simulink model "kinovaMicoSimscapeModel"  (R2021b)
settings: Solver=VariableStepAuto  StartTime=0.0  StopTime=0.3  FixedStep=0.01  RelTol=1e-3
PostLoadFcn:
  | micoRigidBodyTreeCreation;
  | IC=deg2rad([-90,180,180,0,0,0]);
  | interactiveHomePosition=deg2rad([-90 90 177.5 90 0 0]');
  | load("./KinovaMicoSimscapeVariantConfigurations.mat");
values from neighbouring files (symbols this model uses):
  micoCandlePosition = deg2rad([0,180,180,0,0,0])    [KinovaMicoSimscapeInitializeScript.m]    (also in generatingRandomTrajectory.m)
  ViaPointsTaskSpace = [ViaPointsTaskSpace;[[pi;0;pi],[pi;0;pi],[pi;0;pi],[pi;0;pi],[0;0;0],[0;0;0],[pi;0;pi]]]    [KinovaMicoSimscapeInitializeScript.m]    (also in generatingRandomTrajectory.m = [ViaPointsTaskSpace;zeros(3,7)])
undefined symbols (not defined in the file or in its folder): Mico, ViaPointsJointSpace, X, Y, Z
libraries: sm_lib x26, nesl_utility x19, robotcorelib x4, robotmaniplib x3, pid_lib x2
(part 49 of 50)

== matlab function kinovaMicoSimscapeModel/Variant Subsystem/TaskSpaceController/Sliding Robust Task Space Control/dJdt ==
  data: q input; dJdt output; dq input
function dJdt = fcn(q,dq)
q1=q(1);
q2=q(2);
q3=q(3);
q4=q(4);
q5=q(5);

dq1=dq(1);
dq2=dq(2);
dq3=dq(3);
dq4=dq(4);
dq5=dq(5);

dJdt1_1 = 0.14155926623698178445920348167419*sin(q5)*(cos(q4)*(dq1*cos(q1)*cos(q2)*cos(q3) + dq1*cos(q1)*sin(q2)*sin(q3) + dq2*cos(q2)*sin(q1)*sin(q3) - 1.0*dq2*cos(q3)*sin(q1)*sin(q2) - 1.0*dq3*cos(q2)*sin(q1)*sin(q3) + dq3*cos(q3)*sin(q1)*sin(q2)) - 1.0*dq4*sin(q4)*(sin(q1)*sin(q2)*sin(q3) + cos(q2)*cos(q3)*sin(q1)) + dq4*cos(q1)*cos(q4) - 1.0*dq1*sin(q1)*sin(q4)) - 0.14484150251703908907074946910143*sin(q4)*(dq1*cos(q1)*cos(q2)*cos(q3) + dq1*cos(q1)*sin(q2)*sin(q3) + dq2*cos(q2)*sin(q1)*sin(q3) - 1.0*dq2*cos(q3)*sin(q1)*sin(q2) - 1.0*dq3*cos(q2)*sin(q1)*sin(q3) + dq3*cos(q3)*sin(q1)*sin(q2)) - 0.12259392070255614726193016394973*cos(q5)*(dq1*cos(q1)*cos(q2)*sin(q3) - 1.0*dq1*cos(q1)*cos(q3)*sin(q2) - 1.0*dq2*cos(q2)*cos(q3)*sin(q1) + dq3*cos(q2)*cos(q3)*sin(q1) - 1.0*dq2*sin(q1)*sin(q2)*sin(q3) + dq3*sin(q1)*sin(q2)*sin(q3)) + 0.0069999999999996731503415503539145*dq1*sin(q1) + 0.070779633118078777442860882729292*cos(q5)*(sin(q4)*(dq1*cos(q1)*cos(q2)*cos(q3) + dq1*cos(q1)*sin(q2)*sin(q3) + dq2*cos(q2)*sin(q1)*sin(q3) - 1.0*dq2*cos(q3)*sin(q1)*sin(q2) - 1.0*dq3*cos(q2)*sin(q1)*sin(q3) + dq3*cos(q3)*sin(q1)*sin(q2)) + dq1*cos(q4)*sin(q1) + dq4*cos(q1)*sin(q4) + dq4*cos(q4)*(sin(q1)*sin(q2)*sin(q3) + cos(q2)*cos(q3)*sin(q1))) + 0.12259392070255614726193016394973*dq5*sin(q5)*(cos(q2)*sin(q1)*sin(q3) - 1.0*cos(q3)*sin(q1)*sin(q2)) - 0.29000000000002046363078989088535*dq1*cos(q1)*sin(q2) - 0.29000000000002046363078989088535*dq2*cos(q2)*sin(q1) - 0.14484150251703908907074946910143*dq1*cos(q4)*sin(q1) - 0.14484150251703908907074946910143*dq4*cos(q1)*sin(q4) + 0.14155926623698178445920348167419*dq5*cos(q5)*(cos(q1)*sin(q4) + cos(q4)*(sin(q1)*sin(q2)*sin(q3) + cos(q2)*cos(q3)*sin(q1))) + 0.070779633118078777442860882729292*dq5*sin(q5)*(cos(q1)*cos(q4) - 1.0*sin(q4)*(sin(q1)*sin(q2)*sin(q3) + cos(q2)*cos(q3)*sin(q1))) - 0.14484150251703908907074946910143*dq4*cos(q4)*(sin(q1)*sin(q2)*sin(q3) + cos(q2)*cos(q3)*sin(q1)) - 0.24948499999945283889246638864279*dq1*cos(q1)*cos(q2)*sin(q3) + 0.24948499999945283889246638864279*dq1*cos(q1)*cos(q3)*sin(q2) + 0.24948499999945283889246638864279*dq2*cos(q2)*cos(q3)*sin(q1) - 0.24948499999945283889246638864279*dq3*cos(q2)*cos(q3)*sin(q1) + 0.24948499999945283889246638864279*dq2*sin(q1)*sin(q2)*sin(q3) - 0.24948499999945283889246638864279*dq3*sin(q1)*sin(q2)*sin(q3);
dJdt1_2 = 0.12259392070255614726193016394973*cos(q5)*(dq1*cos(q2)*cos(q3)*sin(q1) - 1.0*dq2*cos(q1)*cos(q2)*sin(q3) + dq2*cos(q1)*cos(q3)*sin(q2) + dq3*cos(q1)*cos(q2)*sin(q3) - 1.0*dq3*cos(q1)*cos(q3)*sin(q2) + dq1*sin(q1)*sin(q2)*sin(q3)) - 0.14484150251703908907074946910143*sin(q4)*(dq2*cos(q1)*cos(q2)*cos(q3) - 1.0*dq3*cos(q1)*cos(q2)*cos(q3) + dq1*cos(q2)*sin(q1)*sin(q3) - 1.0*dq1*cos(q3)*sin(q1)*sin(q2) + dq2*cos(q1)*sin(q2)*sin(q3) - 1.0*dq3*cos(q1)*sin(q2)*sin(q3)) + 0.14484150251703908907074946910143*dq4*cos(q4)*(cos(q1)*cos(q2)*sin(q3) - 1.0*cos(q1)*cos(q3)*sin(q2)) + 0.14155926623698178445920348167419*cos(q4)*sin(q5)*(dq2*cos(q1)*cos(q2)*cos(q3) - 1.0*dq3*cos(q1)*cos(q2)*cos(q3) + dq1*cos(q2)*sin(q1)*sin(q3) - 1.0*dq1*cos(q3)*sin(q1)*sin(q2) + dq2*cos(q1)*sin(q2)*sin(q3) - 1.0*dq3*cos(q1)*sin(q2)*sin(q3)) + 0.070779633118078777442860882729292*cos(q5)*sin(q4)*(dq2*cos(q1)*cos(q2)*cos(q3) - 1.0*dq3*cos(q1)*cos(q2)*cos(q3) + dq1*cos(q2)*sin(q1)*sin(q3) - 1.0*dq1*cos(q3)*sin(q1)*sin(q2) + dq2*cos(q1)*sin(q2)*sin(q3) - 1.0*dq3*cos(q1)*sin(q2)*sin(q3)) - 0.29000000000002046363078989088535*dq1*cos(q2)*sin(q1) - 0.29000000000002046363078989088535*dq2*cos(q1)*sin(q2) + 0.12259392070255614726193016394973*dq5*sin(q5)*(cos(q1)*cos(q2)*cos(q3) + cos(q1)*sin(q2)*sin(q3)) + 0.14155926623698178445920348167419*dq4*sin(q4)*sin(q5)*(cos(q1)*cos(q2)*sin(q3) - 1.0*cos(q1)*cos(q3)*sin(q2)) + 0.070779633118078777442860882729292*dq5*sin(q4)*sin(q5)*(cos(q1)*cos(q2)*sin(q3) - 1.0*cos(q1)*cos(q3)*sin(q2)) + 0.24948499999945283889246638864279*dq1*cos(q2)*cos(q3)*sin(q1) - 0.24948499999945283889246638864279*dq2*cos(q1)*cos(q2)*sin(q3) + 0.24948499999945283889246638864279*dq2*cos(q1)*cos(q3)*sin(q2) + 0.24948499999945283889246638864279*dq3*cos(q1)*cos(q2)*sin(q3) - 0.24948499999945283889246638864279*dq3*cos(q1)*cos(q3)*sin(q2) + 0.24948499999945283889246638864279*dq1*sin(q1)*sin(q2)*sin(q3) - 0.070779633118078777442860882729292*dq4*cos(q4)*cos(q5)*(cos(q1)*cos(q2)*sin(q3) - 1.0*cos(q1)*cos(q3)*sin(q2)) - 0.14155926623698178445920348167419*dq5*cos(q4)*cos(q5)*(cos(q1)*cos(q2)*sin(q3) - 1.0*cos(q1)*cos(q3)*sin(q2));
dJdt1_3 = 0.14484150251703908907074946910143*sin(q4)*(dq2*cos(q1)*cos(q2)*cos(q3) - 1.0*dq3*cos(q1)*cos(q2)*cos(q3) + dq1*cos(q2)*sin(q1)*sin(q3) - 1.0*dq1*cos(q3)*sin(q1)*sin(q2) + dq2*cos(q1)*sin(q2)*sin(q3) - 1.0*dq3*cos(q1)*sin(q2)*sin(q3)) - 0.12259392070255614726193016394973*cos(q5)*(dq1*cos(q2)*cos(q3)*sin(q1) - 1.0*dq2*cos(q1)*cos(q2)*sin(q3) + dq2*cos(q1)*cos(q3)*sin(q2) + dq3*cos(q1)*cos(q2)*sin(q3) - 1.0*dq3*cos(q1)*cos(q3)*sin(q2) + dq1*sin(q1)*sin(q2)*sin(q3)) - 0.14484150251703908907074946910143*dq4*cos(q4)*(cos(q1)*cos(q2)*sin(q3) - 1.0*cos(q1)*cos(q3)*sin(q2)) - 0.14155926623698178445920348167419*cos(q4)*sin(q5)*(dq2*cos(q1)*cos(q2)*cos(q3) - 1.0*dq3*cos(q1)*cos(q2)*cos(q3) + dq1*cos(q2)*sin(q1)*sin(q3) - 1.0*dq1*cos(q3)*sin(q1)*sin(q2) + dq2*cos(q1)*sin(q2)*sin(q3) - 1.0*dq3*cos(q1)*sin(q2)*sin(q3)) - 0.070779633118078777442860882729292*cos(q5)*sin(q4)*(dq2*cos(q1)*cos(q2)*cos(q3) - 1.0*dq3*cos(q1)*cos(q2)*cos(q3) + dq1*cos(q2)*sin(q1)*sin(q3) - 1.0*dq1*cos(q3)*sin(q1)*sin(q2) + dq2*cos(q1)*sin(q2)*sin(q3) - 1.0*dq3*cos(q1)*sin(q2)*sin(q3)) - 0.12259392070255614726193016394973*dq5*sin(q5)*(cos(q1)*cos(q2)*cos(q3) + cos(q1)*sin(q2)*sin(q3)) - 0.14155926623698178445920348167419*dq4*sin(q4)*sin(q5)*(cos(q1)*cos(q2)*sin(q3) - 1.0*cos(q1)*cos(q3)*sin(q2)) - 0.070779633118078777442860882729292*dq5*sin(q4)*sin(q5)*(cos(q1)*cos(q2)*sin(q3) - 1.0*cos(q1)*cos(q3)*sin(q2)) - 0.24948499999945283889246638864279*dq1*cos(q2)*cos(q3)*sin(q1) + 0.24948499999945283889246638864279*dq2*cos(q1)*cos(q2)*sin(q3) - 0.24948499999945283889246638864279*dq2*cos(q1)*cos(q3)*sin(q2) - 0.24948499999945283889246638864279*dq3*cos(q1)*cos(q2)*sin(q3) + 0.24948499999945283889246638864279*dq3*cos(q1)*cos(q3)*sin(q2) - 0.24948499999945283889246638864279*dq1*sin(q1)*sin(q2)*sin(q3) + 0.070779633118078777442860882729292*dq4*cos(q4)*cos(q5)*(cos(q1)*cos(q2)*sin(q3) - 1.0*cos(q1)*cos(q3)*sin(q2)) + 0.14155926623698178445920348167419*dq5*cos(q4)*cos(q5)*(cos(q1)*cos(q2)*sin(q3) - 1.0*cos(q1)*cos(q3)*sin(q2));
dJdt1_4 = 0.070779633118078777442860882729292*cos(q5)*(cos(q4)*(dq1*cos(q2)*cos(q3)*sin(q1) - 1.0*dq2*cos(q1)*cos(q2)*sin(q3) + dq2*cos(q1)*cos(q3)*sin(q2) + dq3*cos(q1)*cos(q2)*sin(q3) - 1.0*dq3*cos(q1)*cos(q3)*sin(q2) + dq1*sin(q1)*sin(q2)*sin(q3)) + dq1*cos(q1)*sin(q4) + dq4*cos(q4)*sin(q1) + dq4*sin(q4)*(cos(q1)*cos(q2)*cos(q3) + cos(q1)*sin(q2)*sin(q3))) - 0.14484150251703908907074946910143*cos(q4)*(dq1*cos(q2)*cos(q3)*sin(q1) - 1.0*dq2*cos(q1)*cos(q2)*sin(q3) + dq2*cos(q1)*cos(q3)*sin(q2) + dq3*cos(q1)*cos(q2)*sin(q3) - 1.0*dq3*cos(q1)*cos(q3)*sin(q2) + dq1*sin(q1)*sin(q2)*sin(q3)) - 0.14155926623698178445920348167419*sin(q5)*(sin(q4)*(dq1*cos(q2)*cos(q3)*sin(q1) - 1.0*dq2*cos(q1)*cos(q2)*sin(q3) + dq2*cos(q1)*cos(q3)*sin(q2) + dq3*cos(q1)*cos(q2)*sin(q3) - 1.0*dq3*cos(q1)*cos(q3)*sin(q2) + dq1*sin(q1)*sin(q2)*sin(q3)) - 1.0*dq1*cos(q1)*cos(q4) + dq4*sin(q1)*sin(q4) - 1.0*dq4*cos(q4)*(cos(q1)*cos(q2)*cos(q3) + cos(q1)*sin(q2)*sin(q3))) - 0.14484150251703908907074946910143*dq1*cos(q1)*sin(q4) - 0.14484150251703908907074946910143*dq4*cos(q4)*sin(q1) + 0.14155926623698178445920348167419*dq5*cos(q5)*(cos(q4)*sin(q1) + sin(q4)*(cos(q1)*cos(q2)*cos(q3) + cos(q1)*sin(q2)*sin(q3))) - 0.070779633118078777442860882729292*dq5*sin(q5)*(sin(q1)*sin(q4) - 1.0*cos(q4)*(cos(q1)*cos(q2)*cos(q3) + cos(q1)*sin(q2)*sin(q3))) - 0.14484150251703908907074946910143*dq4*sin(q4)*(cos(q1)*cos(q2)*cos(q3) + cos(q1)*sin(q2)*sin(q3));
dJdt1_5 = 0.12259392070255614726193016394973*sin(q5)*(dq2*cos(q1)*cos(q2)*cos(q3) - 1.0*dq3*cos(q1)*cos(q2)*cos(q3) + dq1*cos(q2)*sin(q1)*sin(q3) - 1.0*dq1*cos(q3)*sin(q1)*sin(q2) + dq2*cos(q1)*sin(q2)*sin(q3) - 1.0*dq3*cos(q1)*sin(q2)*sin(q3)) - 0.070779633118078777442860882729292*sin(q5)*(sin(q4)*(dq1*cos(q2)*cos(q3)*sin(q1) - 1.0*dq2*cos(q1)*cos(q2)*sin(q3) + dq2*cos(q1)*cos(q3)*sin(q2) + dq3*cos(q1)*cos(q2)*sin(q3) - 1.0*dq3*cos(q1)*cos(q3)*sin(q2) + dq1*sin(q1)*sin(q2)*sin(q3)) - 1.0*dq1*cos(q1)*cos(q4) + dq4*sin(q1)*sin(q4) - 1.0*dq4*cos(q4)*(cos(q1)*cos(q2)*cos(q3) + cos(q1)*sin(q2)*sin(q3))) + 0.14155926623698178445920348167419*cos(q5)*(cos(q4)*(dq1*cos(q2)*cos(q3)*sin(q1) - 1.0*dq2*cos(q1)*cos(q2)*sin(q3) + dq2*cos(q1)*cos(q3)*sin(q2) + dq3*cos(q1)*cos(q2)*sin(q3) - 1.0*dq3*cos(q1)*cos(q3)*sin(q2) + dq1*sin(q1)*sin(q2)*sin(q3)) + dq1*cos(q1)*sin(q4) + dq4*cos(q4)*sin(q1) + dq4*sin(q4)*(cos(q1)*cos(q2)*cos(q3) + cos(q1)*sin(q2)*sin(q3))) - 0.12259392070255614726193016394973*dq5*cos(q5)*(cos(q1)*cos(q2)*sin(q3) - 1.0*cos(q1)*cos(q3)*sin(q2)) + 0.070779633118078777442860882729292*dq5*cos(q5)*(cos(q4)*sin(q1) + sin(q4)*(cos(q1)*cos(q2)*cos(q3) + cos(q1)*sin(q2)*sin(q3))) - 0.14155926623698178445920348167419*dq5*sin(q5)*(sin(q1)*sin(q4) - 1.0*cos(q4)*(cos(q1)*cos(q2)*cos(q3) + cos(q1)*sin(q2)*sin(q3)));
dJdt1_6 = 0.0;
dJdt2_1 = 0.14484150251703908907074946910143*sin(q4)*(dq1*cos(q2)*cos(q3)*sin(q1) - 1.0*dq2*cos(q1)*cos(q2)*sin(q3) + dq2*cos(q1)*cos(q3)*sin(q2) + dq3*cos(q1)*cos(q2)*sin(q3) - 1.0*dq3*cos(q1)*cos(q3)*sin(q2) + dq1*sin(q1)*sin(q2)*sin(q3)) - 0.070779633118078777442860882729292*cos(q5)*(sin(q4)*(dq1*cos(q2)*cos(q3)*sin(q1) - 1.0*dq2*cos(q1)*cos(q2)*sin(q3) + dq2*cos(q1)*cos(q3)*sin(q2) + dq3*cos(q1)*cos(q2)*sin(q3) - 1.0*dq3*cos(q1)*cos(q3)*sin(q2) + dq1*sin(q1)*sin(q2)*sin(q3)) - 1.0*dq1*cos(q1)*cos(q4) + dq4*sin(q1)*sin(q4) - 1.0*dq4*cos(q4)*(cos(q1)*cos(q2)*cos(q3) + cos(q1)*sin(q2)*sin(q3))) + 0.12259392070255614726193016394973*cos(q5)*(dq2*cos(q1)*cos(q2)*cos(q3) - 1.0*dq3*cos(q1)*cos(q2)*cos(q3) + dq1*cos(q2)*sin(q1)*sin(q3) - 1.0*dq1*cos(q3)*sin(q1)*sin(q2) + dq2*cos(q1)*sin(q2)*sin(q3) - 1.0*dq3*cos(q1)*sin(q2)*sin(q3)) - 0.14155926623698178445920348167419*sin(q5)*(cos(q4)*(dq1*cos(q2)*cos(q3)*sin(q1) - 1.0*dq2*cos(q1)*cos(q2)*sin(q3) + dq2*cos(q1)*cos(q3)*sin(q2) + dq3*cos(q1)*cos(q2)*sin(q3) - 1.0*dq3*cos(q1)*cos(q3)*sin(q2) + dq1*sin(q1)*sin(q2)*sin(q3)) + dq1*cos(q1)*sin(q4) + dq4*cos(q4)*sin(q1) + dq4*sin(q4)*(cos(q1)*cos(q2)*cos(q3) + cos(q1)*sin(q2)*sin(q3))) + 0.0069999999999996731503415503539145*dq1*cos(q1) + 0.12259392070255614726193016394973*dq5*sin(q5)*(cos(q1)*cos(q2)*sin(q3) - 1.0*cos(q1)*cos(q3)*sin(q2)) - 0.29000000000002046363078989088535*dq2*cos(q1)*cos(q2) - 0.14484150251703908907074946910143*dq1*cos(q1)*cos(q4) + 0.29000000000002046363078989088535*dq1*sin(q1)*sin(q2) + 0.14484150251703908907074946910143*dq4*sin(q1)*sin(q4) - 0.070779633118078777442860882729292*dq5*sin(q5)*(cos(q4)*sin(q1) + sin(q4)*(cos(q1)*cos(q2)*cos(q3) + cos(q1)*sin(q2)*sin(q3))) - 0.14155926623698178445920348167419*dq5*cos(q5)*(sin(q1)*sin(q4) - 1.0*cos(q4)*(cos(q1)*cos(q2)*cos(q3) + cos(q1)*sin(q2)*sin(q3))) - 0.14484150251703908907074946910143*dq4*cos(q4)*(cos(q1)*cos(q2)*cos(q3) + cos(q1)*sin(q2)*sin(q3)) + 0.24948499999945283889246638864279*dq2*cos(q1)*cos(q2)*cos(q3) - 0.24948499999945283889246638864279*dq3*cos(q1)*cos(q2)*cos(q3) + 0.24948499999945283889246638864279*dq1*cos(q2)*sin(q1)*sin(q3) - 0.24948499999945283889246638864279*dq1*cos(q3)*sin(q1)*sin(q2) + 0.24948499999945283889246638864279*dq2*cos(q1)*sin(q2)*sin(q3) - 0.24948499999945283889246638864279*dq3*cos(q1)*sin(q2)*sin(q3);
dJdt2_2 = 0.12259392070255614726193016394973*cos(q5)*(dq1*cos(q1)*cos(q2)*cos(q3) + dq1*cos(q1)*sin(q2)*sin(q3) + dq2*cos(q2)*sin(q1)*sin(q3) - 1.0*dq2*cos(q3)*sin(q1)*sin(q2) - 1.0*dq3*cos(q2)*sin(q1)*sin(q3) + dq3*cos(q3)*sin(q1)*sin(q2)) - 0.14484150251703908907074946910143*sin(q4)*(dq1*cos(q1)*cos(q2)*sin(q3) - 1.0*dq1*cos(q1)*cos(q3)*sin(q2) - 1.0*dq2*cos(q2)*cos(q3)*sin(q1) + dq3*cos(q2)*cos(q3)*sin(q1) - 1.0*dq2*sin(q1)*sin(q2)*sin(q3) + dq3*sin(q1)*sin(q2)*sin(q3)) - 0.12259392070255614726193016394973*dq5*sin(q5)*(sin(q1)*sin(q2)*sin(q3) + cos(q2)*cos(q3)*sin(q1)) - 0.14484150251703908907074946910143*dq4*cos(q4)*(cos(q2)*sin(q1)*sin(q3) - 1.0*cos(q3)*sin(q1)*sin(q2)) + 0.14155926623698178445920348167419*cos(q4)*sin(q5)*(dq1*cos(q1)*cos(q2)*sin(q3) - 1.0*dq1*cos(q1)*cos(q3)*sin(q2) - 1.0*dq2*cos(q2)*cos(q3)*sin(q1) + dq3*cos(q2)*cos(q3)*sin(q1) - 1.0*dq2*sin(q1)*sin(q2)*sin(q3) + dq3*sin(q1)*sin(q2)*sin(q3)) + 0.070779633118078777442860882729292*cos(q5)*sin(q4)*(dq1*cos(q1)*cos(q2)*sin(q3) - 1.0*dq1*cos(q1)*cos(q3)*sin(q2) - 1.0*dq2*cos(q2)*cos(q3)*sin(q1) + dq3*cos(q2)*cos(q3)*sin(q1) - 1.0*dq2*sin(q1)*sin(q2)*sin(q3) + dq3*sin(q1)*sin(q2)*sin(q3)) - 0.29000000000002046363078989088535*dq1*cos(q1)*cos(q2) + 0.29000000000002046363078989088535*dq2*sin(q1)*sin(q2) + 0.070779633118078777442860882729292*dq4*cos(q4)*cos(q5)*(cos(q2)*sin(q1)*sin(q3) - 1.0*cos(q3)*sin(q1)*sin(q2)) + 0.14155926623698178445920348167419*dq5*cos(q4)*cos(q5)*(cos(q2)*sin(q1)*sin(q3) - 1.0*cos(q3)*sin(q1)*sin(q2)) - 0.14155926623698178445920348167419*dq4*sin(q4)*sin(q5)*(cos(q2)*sin(q1)*sin(q3) - 1.0*cos(q3)*sin(q1)*sin(q2)) - 0.070779633118078777442860882729292*dq5*sin(q4)*sin(q5)*(cos(q2)*sin(q1)*sin(q3) - 1.0*cos(q3)*sin(q1)*sin(q2)) + 0.24948499999945283889246638864279*dq1*cos(q1)*cos(q2)*cos(q3) + 0.24948499999945283889246638864279*dq1*cos(q1)*sin(q2)*sin(q3) + 0.24948499999945283889246638864279*dq2*cos(q2)*sin(q1)*sin(q3) - 0.24948499999945283889246638864279*dq2*cos(q3)*sin(q1)*sin(q2) - 0.24948499999945283889246638864279*dq3*cos(q2)*sin(q1)*sin(q3) + 0.24948499999945283889246638864279*dq3*cos(q3)*sin(q1)*sin(q2);
dJdt2_3 = 0.14484150251703908907074946910143*sin(q4)*(dq1*cos(q1)*cos(q2)*sin(q3) - 1.0*dq1*cos(q1)*cos(q3)*sin(q2) - 1.0*dq2*cos(q2)*cos(q3)*sin(q1) + dq3*cos(q2)*cos(q3)*sin(q1) - 1.0*dq2*sin(q1)*sin(q2)*sin(q3) + dq3*sin(q1)*sin(q2)*sin(q3)) - 0.12259392070255614726193016394973*cos(q5)*(dq1*cos(q1)*cos(q2)*cos(q3) + dq1*cos(q1)*sin(q2)*sin(q3) + dq2*cos(q2)*sin(q1)*sin(q3) - 1.0*dq2*cos(q3)*sin(q1)*sin(q2) - 1.0*dq3*cos(q2)*sin(q1)*sin(q3) + dq3*cos(q3)*sin(q1)*sin(q2)) + 0.12259392070255614726193016394973*dq5*sin(q5)*(sin(q1)*sin(q2)*sin(q3) + cos(q2)*cos(q3)*sin(q1)) + 0.14484150251703908907074946910143*dq4*cos(q4)*(cos(q2)*sin(q1)*sin(q3) - 1.0*cos(q3)*sin(q1)*sin(q2)) - 0.14155926623698178445920348167419*cos(q4)*sin(q5)*(dq1*cos(q1)*cos(q2)*sin(q3) - 1.0*dq1*cos(q1)*cos(q3)*sin(q2) - 1.0*dq2*cos(q2)*cos(q3)*sin(q1) + dq3*cos(q2)*cos(q3)*sin(q1) - 1.0*dq2*sin(q1)*sin(q2)*sin(q3) + dq3*sin(q1)*sin(q2)*sin(q3)) - 0.070779633118078777442860882729292*cos(q5)*sin(q4)*(dq1*cos(q1)*cos(q2)*sin(q3) - 1.0*dq1*cos(q1)*cos(q3)*sin(q2) - 1.0*dq2*cos(q2)*cos(q3)*sin(q1) + dq3*cos(q2)*cos(q3)*sin(q1) - 1.0*dq2*sin(q1)*sin(q2)*sin(q3) + dq3*sin(q1)*sin(q2)*sin(q3)) - 0.070779633118078777442860882729292*dq4*cos(q4)*cos(q5)*(cos(q2)*sin(q1)*sin(q3) - 1.0*cos(q3)*sin(q1)*sin(q2)) - 0.14155926623698178445920348167419*dq5*cos(q4)*cos(q5)*(cos(q2)*sin(q1)*sin(q3) - 1.0*cos(q3)*sin(q1)*sin(q2)) + 0.14155926623698178445920348167419*dq4*sin(q4)*sin(q5)*(cos(q2)*sin(q1)*sin(q3) - 1.0*cos(q3)*sin(q1)*sin(q2)) + 0.070779633118078777442860882729292*dq5*sin(q4)*sin(q5)*(cos(q2)*sin(q1)*sin(q3) - 1.0*cos(q3)*sin(q1)*sin(q2)) - 0.24948499999945283889246638864279*dq1*cos(q1)*cos(q2)*cos(q3) - 0.24948499999945283889246638864279*dq1*cos(q1)*sin(q2)*sin(q3) - 0.24948499999945283889246638864279*dq2*cos(q2)*sin(q1)*sin(q3) + 0.24948499999945283889246638864279*dq2*cos(q3)*sin(q1)*sin(q2) + 0.24948499999945283889246638864279*dq3*cos(q2)*sin(q1)*sin(q3) - 0.24948499999945283889246638864279*dq3*cos(q3)*sin(q1)*sin(q2);
dJdt2_4 = 0.070779633118078777442860882729292*cos(q5)*(cos(q4)*(dq1*cos(q1)*cos(q2)*cos(q3) + dq1*cos(q1)*sin(q2)*sin(q3) + dq2*cos(q2)*sin(q1)*sin(q3) - 1.0*dq2*cos(q3)*sin(q1)*sin(q2) - 1.0*dq3*cos(q2)*sin(q1)*sin(q3) + dq3*cos(q3)*sin(q1)*sin(q2)) - 1.0*dq4*sin(q4)*(sin(q1)*sin(q2)*sin(q3) + cos(q2)*cos(q3)*sin(q1)) + dq4*cos(q1)*cos(q4) - 1.0*dq1*sin(q1)*sin(q4)) - 0.14484150251703908907074946910143*cos(q4)*(dq1*cos(q1)*cos(q2)*cos(q3) + dq1*cos(q1)*sin(q2)*sin(q3) + dq2*cos(q2)*sin(q1)*sin(q3) - 1.0*dq2*cos(q3)*sin(q1)*sin(q2) - 1.0*dq3*cos(q2)*sin(q1)*sin(q3) + dq3*cos(q3)*sin(q1)*sin(q2)) - 0.14155926623698178445920348167419*sin(q5)*(sin(q4)*(dq1*cos(q1)*cos(q2)*cos(q3) + dq1*cos(q1)*sin(q2)*sin(q3) + dq2*cos(q2)*sin(q1)*sin(q3) - 1.0*dq2*cos(q3)*sin(q1)*sin(q2) - 1.0*dq3*cos(q2)*sin(q1)*sin(q3) + dq3*cos(q3)*sin(q1)*sin(q2)) + dq1*cos(q4)*sin(q1) + dq4*cos(q1)*sin(q4) + dq4*cos(q4)*(sin(q1)*sin(q2)*sin(q3) + cos(q2)*cos(q3)*sin(q1))) + 0.14484150251703908907074946910143*dq4*sin(q4)*(sin(q1)*sin(q2)*sin(q3) + cos(q2)*cos(q3)*sin(q1)) - 0.14484150251703908907074946910143*dq4*cos(q1)*cos(q4) + 0.14484150251703908907074946910143*dq1*sin(q1)*sin(q4) - 0.070779633118078777442860882729292*dq5*sin(q5)*(cos(q1)*sin(q4) + cos(q4)*(sin(q1)*sin(q2)*sin(q3) + cos(q2)*cos(q3)*sin(q1))) + 0.14155926623698178445920348167419*dq5*cos(q5)*(cos(q1)*cos(q4) - 1.0*sin(q4)*(sin(q1)*sin(q2)*sin(q3) + cos(q2)*cos(q3)*sin(q1)));
dJdt2_5 = 0.14155926623698178445920348167419*cos(q5)*(cos(q4)*(dq1*cos(q1)*cos(q2)*cos(q3) + dq1*cos(q1)*sin(q2)*sin(q3) + dq2*cos(q2)*sin(q1)*sin(q3) - 1.0*dq2*cos(q3)*sin(q1)*sin(q2) - 1.0*dq3*cos(q2)*sin(q1)*sin(q3) + dq3*cos(q3)*sin(q1)*sin(q2)) - 1.0*dq4*sin(q4)*(sin(q1)*sin(q2)*sin(q3) + cos(q2)*cos(q3)*sin(q1)) + dq4*cos(q1)*cos(q4) - 1.0*dq1*sin(q1)*sin(q4)) + 0.12259392070255614726193016394973*sin(q5)*(dq1*cos(q1)*cos(q2)*sin(q3) - 1.0*dq1*cos(q1)*cos(q3)*sin(q2) - 1.0*dq2*cos(q2)*cos(q3)*sin(q1) + dq3*cos(q2)*cos(q3)*sin(q1) - 1.0*dq2*sin(q1)*sin(q2)*sin(q3) + dq3*sin(q1)*sin(q2)*sin(q3)) - 0.070779633118078777442860882729292*sin(q5)*(sin(q4)*(dq1*cos(q1)*cos(q2)*cos(q3) + dq1*cos(q1)*sin(q2)*sin(q3) + dq2*cos(q2)*sin(q1)*sin(q3) - 1.0*dq2*cos(q3)*sin(q1)*sin(q2) - 1.0*dq3*cos(q2)*sin(q1)*sin(q3) + dq3*cos(q3)*sin(q1)*sin(q2)) + dq1*cos(q4)*sin(q1) + dq4*cos(q1)*sin(q4) + dq4*cos(q4)*(sin(q1)*sin(q2)*sin(q3) + cos(q2)*cos(q3)*sin(q1))) + 0.12259392070255614726193016394973*dq5*cos(q5)*(cos(q2)*sin(q1)*sin(q3) - 1.0*cos(q3)*sin(q1)*sin(q2)) - 0.14155926623698178445920348167419*dq5*sin(q5)*(cos(q1)*sin(q4) + cos(q4)*(sin(q1)*sin(q2)*sin(q3) + cos(q2)*cos(q3)*sin(q1))) + 0.070779633118078777442860882729292*dq5*cos(q5)*(cos(q1)*cos(q4) - 1.0*sin(q4)*(sin(q1)*sin(q2)*sin(q3) + cos(q2)*cos(q3)*sin(q1)));
dJdt2_6 = 0.0;
dJdt3_1 = 0.0;
dJdt3_2 = 0.14484150251703908907074946910143*sin(q4)*(dq2*cos(q2)*sin(q3) - 1.0*dq2*cos(q3)*sin(q2) - 1.0*dq3*cos(q2)*sin(q3) + dq3*cos(q3)*sin(q2)) - 0.12259392070255614726193016394973*cos(q5)*(dq2*cos(q2)*cos(q3) - 1.0*dq3*cos(q2)*cos(q3) + dq2*sin(q2)*sin(q3) - 1.0*dq3*sin(q2)*sin(q3)) + 0.29000000000002046363078989088535*dq2*cos(q2) + 0.14484150251703908907074946910143*dq4*cos(q4)*(cos(q2)*cos(q3) + sin(q2)*sin(q3)) - 0.24948499999945283889246638864279*dq2*cos(q2)*cos(q3) + 0.24948499999945283889246638864279*dq3*cos(q2)*cos(q3) - 0.12259392070255614726193016394973*dq5*sin(q5)*(cos(q2)*sin(q3) - 1.0*cos(q3)*sin(q2)) - 0.24948499999945283889246638864279*dq2*sin(q2)*sin(q3) + 0.24948499999945283889246638864279*dq3*sin(q2)*sin(q3) - 0.14155926623698178445920348167419*cos(q4)*sin(q5)*(dq2*cos(q2)*sin(q3) - 1.0*dq2*cos(q3)*sin(q2) - 1.0*dq3*cos(q2)*sin(q3) + dq3*cos(q3)*sin(q2)) - 0.070779633118078777442860882729292*cos(q5)*sin(q4)*(dq2*cos(q2)*sin(q3) - 1.0*dq2*cos(q3)*sin(q2) - 1.0*dq3*cos(q2)*sin(q3) + dq3*cos(q3)*sin(q2)) + 0.14155926623698178445920348167419*dq4*sin(q4)*sin(q5)*(cos(q2)*cos(q3) + sin(q2)*sin(q3)) + 0.070779633118078777442860882729292*dq5*sin(q4)*sin(q5)*(cos(q2)*cos(q3) + sin(q2)*sin(q3)) - 0.070779633118078777442860882729292*dq4*cos(q4)*cos(q5)*(cos(q2)*cos(q3) + sin(q2)*sin(q3)) - 0.14155926623698178445920348167419*dq5*cos(q4)*cos(q5)*(cos(q2)*cos(q3) + sin(q2)*sin(q3));
dJdt3_3 = 0.12259392070255614726193016394973*cos(q5)*(dq2*cos(q2)*cos(q3) - 1.0*dq3*cos(q2)*cos(q3) + dq2*sin(q2)*sin(q3) - 1.0*dq3*sin(q2)*sin(q3)) - 0.14484150251703908907074946910143*sin(q4)*(dq2*cos(q2)*sin(q3) - 1.0*dq2*cos(q3)*sin(q2) - 1.0*dq3*cos(q2)*sin(q3) + dq3*cos(q3)*sin(q2)) - 0.14484150251703908907074946910143*dq4*cos(q4)*(cos(q2)*cos(q3) + sin(q2)*sin(q3)) + 0.24948499999945283889246638864279*dq2*cos(q2)*cos(q3) - 0.24948499999945283889246638864279*dq3*cos(q2)*cos(q3) + 0.12259392070255614726193016394973*dq5*sin(q5)*(cos(q2)*sin(q3) - 1.0*cos(q3)*sin(q2)) + 0.24948499999945283889246638864279*dq2*sin(q2)*sin(q3) - 0.24948499999945283889246638864279*dq3*sin(q2)*sin(q3) + 0.14155926623698178445920348167419*cos(q4)*sin(q5)*(dq2*cos(q2)*sin(q3) - 1.0*dq2*cos(q3)*sin(q2) - 1.0*dq3*cos(q2)*sin(q3) + dq3*cos(q3)*sin(q2)) + 0.070779633118078777442860882729292*cos(q5)*sin(q4)*(dq2*cos(q2)*sin(q3) - 1.0*dq2*cos(q3)*sin(q2) - 1.0*dq3*cos(q2)*sin(q3) + dq3*cos(q3)*sin(q2)) - 0.14155926623698178445920348167419*dq4*sin(q4)*sin(q5)*(cos(q2)*cos(q3) + sin(q2)*sin(q3)) - 0.070779633118078777442860882729292*dq5*sin(q4)*sin(q5)*(cos(q2)*cos(q3) + sin(q2)*sin(q3)) + 0.070779633118078777442860882729292*dq4*cos(q4)*cos(q5)*(cos(q2)*cos(q3) + sin(q2)*sin(q3)) + 0.14155926623698178445920348167419*dq5*cos(q4)*cos(q5)*(cos(q2)*cos(q3) + sin(q2)*sin(q3));
dJdt3_4 = 0.14484150251703908907074946910143*cos(q4)*(dq2*cos(q2)*cos(q3) - 1.0*dq3*cos(q2)*cos(q3) + dq2*sin(q2)*sin(q3) - 1.0*dq3*sin(q2)*sin(q3)) + 0.14484150251703908907074946910143*dq4*sin(q4)*(cos(q2)*sin(q3) - 1.0*cos(q3)*sin(q2)) - 0.070779633118078777442860882729292*cos(q4)*cos(q5)*(dq2*cos(q2)*cos(q3) - 1.0*dq3*cos(q2)*cos(q3) + dq2*sin(q2)*sin(q3) - 1.0*dq3*sin(q2)*sin(q3)) + 0.14155926623698178445920348167419*sin(q4)*sin(q5)*(dq2*cos(q2)*cos(q3) - 1.0*dq3*cos(q2)*cos(q3) + dq2*sin(q2)*sin(q3) - 1.0*dq3*sin(q2)*sin(q3)) - 0.14155926623698178445920348167419*dq4*cos(q4)*sin(q5)*(cos(q2)*sin(q3) - 1.0*cos(q3)*sin(q2)) - 0.070779633118078777442860882729292*dq4*cos(q5)*sin(q4)*(cos(q2)*sin(q3) - 1.0*cos(q3)*sin(q2)) - 0.070779633118078777442860882729292*dq5*cos(q4)*sin(q5)*(cos(q2)*sin(q3) - 1.0*cos(q3)*sin(q2)) - 0.14155926623698178445920348167419*dq5*cos(q5)*sin(q4)*(cos(q2)*sin(q3) - 1.0*cos(q3)*sin(q2));
dJdt3_5 = 0.070779633118078777442860882729292*sin(q4)*sin(q5)*(dq2*cos(q2)*cos(q3) - 1.0*dq3*cos(q2)*cos(q3) + dq2*sin(q2)*sin(q3) - 1.0*dq3*sin(q2)*sin(q3)) - 0.12259392070255614726193016394973*dq5*cos(q5)*(cos(q2)*cos(q3) + sin(q2)*sin(q3)) - 0.14155926623698178445920348167419*cos(q4)*cos(q5)*(dq2*cos(q2)*cos(q3) - 1.0*dq3*cos(q2)*cos(q3) + dq2*sin(q2)*sin(q3) - 1.0*dq3*sin(q2)*sin(q3)) - 0.12259392070255614726193016394973*sin(q5)*(dq2*cos(q2)*sin(q3) - 1.0*dq2*cos(q3)*sin(q2) - 1.0*dq3*cos(q2)*sin(q3) + dq3*cos(q3)*sin(q2)) - 0.070779633118078777442860882729292*dq4*cos(q4)*sin(q5)*(cos(q2)*sin(q3) - 1.0*cos(q3)*sin(q2)) - 0.14155926623698178445920348167419*dq4*cos(q5)*sin(q4)*(cos(q2)*sin(q3) - 1.0*cos(q3)*sin(q2)) - 0.14155926623698178445920348167419*dq5*cos(q4)*sin(q5)*(cos(q2)*sin(q3) - 1.0*cos(q3)*sin(q2)) - 0.070779633118078777442860882729292*dq5*cos(q5)*sin(q4)*(cos(q2)*sin(q3) - 1.0*cos(q3)*sin(q2));
dJdt3_6 = 0.0;
dJdt4_1 = 0.0;
dJdt4_2 = -1.0*dq1*cos(q1);
dJdt4_3 = dq1*cos(q1);
dJdt4_4 = dq2*cos(q1)*cos(q2)*cos(q3) - 1.0*dq3*cos(q1)*cos(q2)*cos(q3) + dq1*cos(q2)*sin(q1)*sin(q3) - 1.0*dq1*cos(q3)*sin(q1)*sin(q2) + dq2*cos(q1)*sin(q2)*sin(q3) - 1.0*dq3*cos(q1)*sin(q2)*sin(q3);
dJdt4_5 = 0.86602540378612502536270767450333*sin(q4)*(dq1*cos(q2)*cos(q3)*sin(q1) - 1.0*dq2*cos(q1)*cos(q2)*sin(q3) + dq2*cos(q1)*cos(q3)*sin(q2) + dq3*cos(q1)*cos(q2)*sin(q3) - 1.0*dq3*cos(q1)*cos(q3)*sin(q2) + dq1*sin(q1)*sin(q2)*sin(q3)) - 0.86602540378612502536270767450333*dq1*cos(q1)*cos(q4) + 0.86602540378612502536270767450333*dq4*sin(q1)*sin(q4) - 0.86602540378612502536270767450333*dq4*cos(q4)*(cos(q1)*cos(q2)*cos(q3) + cos(q1)*sin(q2)*sin(q3)) + 0.49999999999704414221923798322678*dq2*cos(q1)*cos(q2)*cos(q3) - 0.49999999999704414221923798322678*dq3*cos(q1)*cos(q2)*cos(q3) + 0.49999999999704414221923798322678*dq1*cos(q2)*sin(q1)*sin(q3) - 0.49999999999704414221923798322678*dq1*cos(q3)*sin(q1)*sin(q2) + 0.49999999999704414221923798322678*dq2*cos(q1)*sin(q2)*sin(q3) - 0.49999999999704414221923798322678*dq3*cos(q1)*sin(q2)*sin(q3);
dJdt4_6 = 0.43301270189050455883261747658253*sin(q4)*(dq1*cos(q2)*cos(q3)*sin(q1) - 1.0*dq2*cos(q1)*cos(q2)*sin(q3) + dq2*cos(q1)*cos(q3)*sin(q2) + dq3*cos(q1)*cos(q2)*sin(q3) - 1.0*dq3*cos(q1)*cos(q3)*sin(q2) + dq1*sin(q1)*sin(q2)*sin(q3)) - 0.43301270189050455883261747658253*cos(q5)*(sin(q4)*(dq1*cos(q2)*cos(q3)*sin(q1) - 1.0*dq2*cos(q1)*cos(q2)*sin(q3) + dq2*cos(q1)*cos(q3)*sin(q2) + dq3*cos(q1)*cos(q2)*sin(q3) - 1.0*dq3*cos(q1)*cos(q3)*sin(q2) + dq1*sin(q1)*sin(q2)*sin(q3)) - 1.0*dq1*cos(q1)*cos(q4) + dq4*sin(q1)*sin(q4) - 1.0*dq4*cos(q4)*(cos(q1)*cos(q2)*cos(q3) + cos(q1)*sin(q2)*sin(q3))) + 0.75000000000295585778076201677322*cos(q5)*(dq2*cos(q1)*cos(q2)*cos(q3) - 1.0*dq3*cos(q1)*cos(q2)*cos(q3) + dq1*cos(q2)*sin(q1)*sin(q3) - 1.0*dq1*cos(q3)*sin(q1)*sin(q2) + dq2*cos(q1)*sin(q2)*sin(q3) - 1.0*dq3*cos(q1)*sin(q2)*sin(q3)) - 0.86602540378612502536270767450333*sin(q5)*(cos(q4)*(dq1*cos(q2)*cos(q3)*sin(q1) - 1.0*dq2*cos(q1)*cos(q2)*sin(q3) + dq2*cos(q1)*cos(q3)*sin(q2) + dq3*cos(q1)*cos(q2)*sin(q3) - 1.0*dq3*cos(q1)*cos(q3)*sin(q2) + dq1*sin(q1)*sin(q2)*sin(q3)) + dq1*cos(q1)*sin(q4) + dq4*cos(q4)*sin(q1) + dq4*sin(q4)*(cos(q1)*cos(q2)*cos(q3) + cos(q1)*sin(q2)*sin(q3))) + 0.75000000000295585778076201677322*dq5*sin(q5)*(cos(q1)*cos(q2)*sin(q3) - 1.0*cos(q1)*cos(q3)*sin(q2)) - 0.43301270189050455883261747658253*dq1*cos(q1)*cos(q4) + 0.43301270189050455883261747658253*dq4*sin(q1)*sin(q4) - 0.43301270189050455883261747658253*dq5*sin(q5)*(cos(q4)*sin(q1) + sin(q4)*(cos(q1)*cos(q2)*cos(q3) + cos(q1)*sin(q2)*sin(q3))) - 0.86602540378612502536270767450333*dq5*cos(q5)*(sin(q1)*sin(q4) - 1.0*cos(q4)*(cos(q1)*cos(q2)*cos(q3) + cos(q1)*sin(q2)*sin(q3))) - 0.43301270189050455883261747658253*dq4*cos(q4)*(cos(q1)*cos(q2)*cos(q3) + cos(q1)*sin(q2)*sin(q3)) + 0.24999999999704414221923798322678*dq2*cos(q1)*cos(q2)*cos(q3) - 0.24999999999704414221923798322678*dq3*cos(q1)*cos(q2)*cos(q3) + 0.24999999999704414221923798322678*dq1*cos(q2)*sin(q1)*sin(q3) - 0.24999999999704414221923798322678*dq1*cos(q3)*sin(q1)*sin(q2) + 0.24999999999704414221923798322678*dq2*cos(q1)*sin(q2)*sin(q3) - 0.24999999999704414221923798322678*dq3*cos(q1)*sin(q2)*sin(q3);
dJdt5_1 = 0.0;
dJdt5_2 = dq1*sin(q1);
dJdt5_3 = -1.0*dq1*sin(q1);
dJdt5_4 = dq1*cos(q1)*cos(q2)*sin(q3) - 1.0*dq1*cos(q1)*cos(q3)*sin(q2) - 1.0*dq2*cos(q2)*cos(q3)*sin(q1) + dq3*cos(q2)*cos(q3)*sin(q1) - 1.0*dq2*sin(q1)*sin(q2)*sin(q3) + dq3*sin(q1)*sin(q2)*sin(q3);
dJdt5_5 = 0.86602540378612502536270767450333*sin(q4)*(dq1*cos(q1)*cos(q2)*cos(q3) + dq1*cos(q1)*sin(q2)*sin(q3) + dq2*cos(q2)*sin(q1)*sin(q3) - 1.0*dq2*cos(q3)*sin(q1)*sin(q2) - 1.0*dq3*cos(q2)*sin(q1)*sin(q3) + dq3*cos(q3)*sin(q1)*sin(q2)) + 0.86602540378612502536270767450333*dq1*cos(q4)*sin(q1) + 0.86602540378612502536270767450333*dq4*cos(q1)*sin(q4) + 0.86602540378612502536270767450333*dq4*cos(q4)*(sin(q1)*sin(q2)*sin(q3) + cos(q2)*cos(q3)*sin(q1)) + 0.49999999999704414221923798322678*dq1*cos(q1)*cos(q2)*sin(q3) - 0.49999999999704414221923798322678*dq1*cos(q1)*cos(q3)*sin(q2) - 0.49999999999704414221923798322678*dq2*cos(q2)*cos(q3)*sin(q1) + 0.49999999999704414221923798322678*dq3*cos(q2)*cos(q3)*sin(q1) - 0.49999999999704414221923798322678*dq2*sin(q1)*sin(q2)*sin(q3) + 0.49999999999704414221923798322678*dq3*sin(q1)*sin(q2)*sin(q3);
dJdt5_6 = 0.43301270189050455883261747658253*sin(q4)*(dq1*cos(q1)*cos(q2)*cos(q3) + dq1*cos(q1)*sin(q2)*sin(q3) + dq2*cos(q2)*sin(q1)*sin(q3) - 1.0*dq2*cos(q3)*sin(q1)*sin(q2) - 1.0*dq3*cos(q2)*sin(q1)*sin(q3) + dq3*cos(q3)*sin(q1)*sin(q2)) - 0.86602540378612502536270767450333*sin(q5)*(cos(q4)*(dq1*cos(q1)*cos(q2)*cos(q3) + dq1*cos(q1)*sin(q2)*sin(q3) + dq2*cos(q2)*sin(q1)*sin(q3) - 1.0*dq2*cos(q3)*sin(q1)*sin(q2) - 1.0*dq3*cos(q2)*sin(q1)*sin(q3) + dq3*cos(q3)*sin(q1)*sin(q2)) - 1.0*dq4*sin(q4)*(sin(q1)*sin(q2)*sin(q3) + cos(q2)*cos(q3)*sin(q1)) + dq4*cos(q1)*cos(q4) - 1.0*dq1*sin(q1)*sin(q4)) + 0.75000000000295585778076201677322*cos(q5)*(dq1*cos(q1)*cos(q2)*sin(q3) - 1.0*dq1*cos(q1)*cos(q3)*sin(q2) - 1.0*dq2*cos(q2)*cos(q3)*sin(q1) + dq3*cos(q2)*cos(q3)*sin(q1) - 1.0*dq2*sin(q1)*sin(q2)*sin(q3) + dq3*sin(q1)*sin(q2)*sin(q3)) - 0.43301270189050455883261747658253*cos(q5)*(sin(q4)*(dq1*cos(q1)*cos(q2)*cos(q3) + dq1*cos(q1)*sin(q2)*sin(q3) + dq2*cos(q2)*sin(q1)*sin(q3) - 1.0*dq2*cos(q3)*sin(q1)*sin(q2) - 1.0*dq3*cos(q2)*sin(q1)*sin(q3) + dq3*cos(q3)*sin(q1)*sin(q2)) + dq1*cos(q4)*sin(q1) + dq4*cos(q1)*sin(q4) + dq4*cos(q4)*(sin(q1)*sin(q2)*sin(q3) + cos(q2)*cos(q3)*sin(q1))) - 0.75000000000295585778076201677322*dq5*sin(q5)*(cos(q2)*sin(q1)*sin(q3) - 1.0*cos(q3)*sin(q1)*sin(q2)) + 0.43301270189050455883261747658253*dq1*cos(q4)*sin(q1) + 0.43301270189050455883261747658253*dq4*cos(q1)*sin(q4) - 0.86602540378612502536270767450333*dq5*cos(q5)*(cos(q1)*sin(q4) + cos(q4)*(sin(q1)*sin(q2)*sin(q3) + cos(q2)*cos(q3)*sin(q1))) - 0.43301270189050455883261747658253*dq5*sin(q5)*(cos(q1)*cos(q4) - 1.0*sin(q4)*(sin(q1)*sin(q2)*sin(q3) + cos(q2)*cos(q3)*sin(q1))) + 0.43301270189050455883261747658253*dq4*cos(q4)*(sin(q1)*sin(q2)*sin(q3) + cos(q2)*cos(q3)*sin(q1)) + 0.24999999999704414221923798322678*dq1*cos(q1)*cos(q2)*sin(q3) - 0.24999999999704414221923798322678*dq1*cos(q1)*cos(q3)*sin(q2) - 0.24999999999704414221923798322678*dq2*cos(q2)*cos(q3)*sin(q1) + 0.24999999999704414221923798322678*dq3*cos(q2)*cos(q3)*sin(q1) - 0.24999999999704414221923798322678*dq2*sin(q1)*sin(q2)*sin(q3) + 0.24999999999704414221923798322678*dq3*sin(q1)*sin(q2)*sin(q3);
dJdt6_1 = 0.0;
dJdt6_2 = 0.0;
dJdt6_3 = 0.0;
dJdt6_4 = dq2*cos(q3)*sin(q2) - 1.0*dq2*cos(q2)*sin(q3) + dq3*cos(q2)*sin(q3) - 1.0*dq3*cos(q3)*sin(q2);
dJdt6_5 = 0.86602540378612502536270767450333*dq4*cos(q4)*(cos(q2)*sin(q3) - 1.0*cos(q3)*sin(q2)) - 0.86602540378612502536270767450333*sin(q4)*(dq2*cos(q2)*cos(q3) - 1.0*dq3*cos(q2)*cos(q3) + dq2*sin(q2)*sin(q3) - 1.0*dq3*sin(q2)*sin(q3)) - 0.49999999999704414221923798322678*dq2*cos(q2)*sin(q3) + 0.49999999999704414221923798322678*dq2*cos(q3)*sin(q2) + 0.49999999999704414221923798322678*dq3*cos(q2)*sin(q3) - 0.49999999999704414221923798322678*dq3*cos(q3)*sin(q2);
dJdt6_6 = 0.75000000000295585778076201677322*dq5*sin(q5)*(cos(q2)*cos(q3) + sin(q2)*sin(q3)) - 0.43301270189050455883261747658253*sin(q4)*(dq2*cos(q2)*cos(q3) - 1.0*dq3*cos(q2)*cos(q3) + dq2*sin(q2)*sin(q3) - 1.0*dq3*sin(q2)*sin(q3)) - 0.75000000000295585778076201677322*cos(q5)*(dq2*cos(q2)*sin(q3) - 1.0*dq2*cos(q3)*sin(q2) - 1.0*dq3*cos(q2)*sin(q3) + dq3*cos(q3)*sin(q2)) + 0.43301270189050455883261747658253*dq4*cos(q4)*(cos(q2)*sin(q3) - 1.0*cos(q3)*sin(q2)) - 0.24999999999704414221923798322678*dq2*cos(q2)*sin(q3) + 0.24999999999704414221923798322678*dq2*cos(q3)*sin(q2) + 0.24999999999704414221923798322678*dq3*cos(q2)*sin(q3) - 0.24999999999704414221923798322678*dq3*cos(q3)*sin(q2) + 0.86602540378612502536270767450333*cos(q4)*sin(q5)*(dq2*cos(q2)*cos(q3) - 1.0*dq3*cos(q2)*cos(q3) + dq2*sin(q2)*sin(q3) - 1.0*dq3*sin(q2)*sin(q3)) + 0.43301270189050455883261747658253*cos(q5)*sin(q4)*(dq2*cos(q2)*cos(q3) - 1.0*dq3*cos(q2)*cos(q3) + dq2*sin(q2)*sin(q3) - 1.0*dq3*sin(q2)*sin(q3)) - 0.43301270189050455883261747658253*dq4*cos(q4)*cos(q5)*(cos(q2)*sin(q3) - 1.0*cos(q3)*sin(q2)) - 0.86602540378612502536270767450333*dq5*cos(q4)*cos(q5)*(cos(q2)*sin(q3) - 1.0*cos(q3)*sin(q2)) + 0.86602540378612502536270767450333*dq4*sin(q4)*sin(q5)*(cos(q2)*sin(q3) - 1.0*cos(q3)*sin(q2)) + 0.43301270189050455883261747658253*dq5*sin(q4)*sin(q5)*(cos(q2)*sin(q3) - 1.0*cos(q3)*sin(q2));
 
dJdt = [dJdt1_1, dJdt1_2, dJdt1_3, dJdt1_4, dJdt1_5, dJdt1_6;
        dJdt2_1, dJdt2_2, dJdt2_3, dJdt2_4, dJdt2_5, dJdt2_6;
        dJdt3_1, dJdt3_2, dJdt3_3, dJdt3_4, dJdt3_5, dJdt3_6;
        dJdt4_1, dJdt4_2, dJdt4_3, dJdt4_4, dJdt4_5, dJdt4_6;
        dJdt5_1, dJdt5_2, dJdt5_3, dJdt5_4, dJdt5_5, dJdt5_6;
        dJdt6_1, dJdt6_2, dJdt6_3, dJdt6_4, dJdt6_5, dJdt6_6];

== stateflow chart kinovaMicoSimscapeModel/Control Logic ==
  state FollowProvidedTrajectory [group]
    state Startup
      engageSelectedController=0;
      trajectorySelector=0;
    state MovingToStartPosition
      engageSelectedController=0;
      trajectorySelector=0;
    state BeginProvidedTrajectory
      trajectorySelector=2;
      engageSelectedController=1;
    (default) -> Startup
    Startup -> MovingToStartPosition
    MovingToStartPosition -> BeginProvidedTrajectory : [q_error<10]
  data: q_error input; dq_error input; trajectorySelector output; engageSelectedController output

== matlab function kinovaMicoSimscapeModel/Variant Subsystem/TaskSpaceController/Inverse Dynamics/MicoJac ==
  data: q input; Jac output
function Jac = fcn(q)
%#codegen
q1=q(1);
q2=q(2);
q3=q(3);
q4=q(4);
q5=q(5);
q6=q(6);


J1_1 = 0.14615*cos(q1)*cos(q4) - 0.007*cos(q1) - 0.29*sin(q1)*sin(q2) + 0.14418*sin(q5)*(cos(q1)*sin(q4) + cos(q4)*(sin(q1)*sin(q2)*sin(q3) + cos(q2)*cos(q3)*sin(q1))) - 0.072089*cos(q5)*(cos(q1)*cos(q4) - 1.0*sin(q4)*(sin(q1)*sin(q2)*sin(q3) + cos(q2)*cos(q3)*sin(q1))) - 0.14615*sin(q4)*(sin(q1)*sin(q2)*sin(q3) + cos(q2)*cos(q3)*sin(q1)) - 0.12486*cos(q5)*(cos(q2)*sin(q1)*sin(q3) - 1.0*cos(q3)*sin(q1)*sin(q2)) - 0.25024*cos(q2)*sin(q1)*sin(q3) + 0.25024*cos(q3)*sin(q1)*sin(q2);
 
J1_2 = 0.29*cos(q1)*cos(q2) - 0.12486*cos(q5)*(cos(q1)*cos(q2)*cos(q3) + cos(q1)*sin(q2)*sin(q3)) + 0.14615*sin(q4)*(cos(q1)*cos(q2)*sin(q3) - 1.0*cos(q1)*cos(q3)*sin(q2)) - 0.14418*cos(q4)*sin(q5)*(cos(q1)*cos(q2)*sin(q3) - 1.0*cos(q1)*cos(q3)*sin(q2)) - 0.072089*cos(q5)*sin(q4)*(cos(q1)*cos(q2)*sin(q3) - 1.0*cos(q1)*cos(q3)*sin(q2)) - 0.25024*cos(q1)*cos(q2)*cos(q3) - 0.25024*cos(q1)*sin(q2)*sin(q3);
 
J1_3 = 0.12486*cos(q5)*(cos(q1)*cos(q2)*cos(q3) + cos(q1)*sin(q2)*sin(q3)) - 0.14615*sin(q4)*(cos(q1)*cos(q2)*sin(q3) - 1.0*cos(q1)*cos(q3)*sin(q2)) + 0.14418*cos(q4)*sin(q5)*(cos(q1)*cos(q2)*sin(q3) - 1.0*cos(q1)*cos(q3)*sin(q2)) + 0.072089*cos(q5)*sin(q4)*(cos(q1)*cos(q2)*sin(q3) - 1.0*cos(q1)*cos(q3)*sin(q2)) + 0.25024*cos(q1)*cos(q2)*cos(q3) + 0.25024*cos(q1)*sin(q2)*sin(q3);
 
J1_4 = 0.14418*sin(q5)*(cos(q4)*sin(q1) + sin(q4)*(cos(q1)*cos(q2)*cos(q3) + cos(q1)*sin(q2)*sin(q3))) - 0.14615*sin(q1)*sin(q4) + 0.072089*cos(q5)*(sin(q1)*sin(q4) - 1.0*cos(q4)*(cos(q1)*cos(q2)*cos(q3) + cos(q1)*sin(q2)*sin(q3))) + 0.14615*cos(q4)*(cos(q1)*cos(q2)*cos(q3) + cos(q1)*sin(q2)*sin(q3));
 
J1_5 = 0.072089*sin(q5)*(cos(q4)*sin(q1) + sin(q4)*(cos(q1)*cos(q2)*cos(q3) + cos(q1)*sin(q2)*sin(q3))) + 0.14418*cos(q5)*(sin(q1)*sin(q4) - 1.0*cos(q4)*(cos(q1)*cos(q2)*cos(q3) + cos(q1)*sin(q2)*sin(q3))) - 0.12486*sin(q5)*(cos(q1)*cos(q2)*sin(q3) - 1.0*cos(q1)*cos(q3)*sin(q2));
 
J1_6 = 0.0;
 
J2_1 = 0.007*sin(q1) - 0.29*cos(q1)*sin(q2) - 0.14615*cos(q4)*sin(q1) + 0.072089*cos(q5)*(cos(q4)*sin(q1) + sin(q4)*(cos(q1)*cos(q2)*cos(q3) + cos(q1)*sin(q2)*sin(q3))) - 0.14418*sin(q5)*(sin(q1)*sin(q4) - 1.0*cos(q4)*(cos(q1)*cos(q2)*cos(q3) + cos(q1)*sin(q2)*sin(q3))) - 0.14615*sin(q4)*(cos(q1)*cos(q2)*cos(q3) + cos(q1)*sin(q2)*sin(q3)) - 0.12486*cos(q5)*(cos(q1)*cos(q2)*sin(q3) - 1.0*cos(q1)*cos(q3)*sin(q2)) - 0.25024*cos(q1)*cos(q2)*sin(q3) + 0.25024*cos(q1)*cos(q3)*sin(q2);
 
J2_2 = 0.12486*cos(q5)*(sin(q1)*sin(q2)*sin(q3) + cos(q2)*cos(q3)*sin(q1)) - 0.29*cos(q2)*sin(q1) - 0.14615*sin(q4)*(cos(q2)*sin(q1)*sin(q3) - 1.0*cos(q3)*sin(q1)*sin(q2)) + 0.25024*sin(q1)*sin(q2)*sin(q3) + 0.14418*cos(q4)*sin(q5)*(cos(q2)*sin(q1)*sin(q3) - 1.0*cos(q3)*sin(q1)*sin(q2)) + 0.072089*cos(q5)*sin(q4)*(cos(q2)*sin(q1)*sin(q3) - 1.0*cos(q3)*sin(q1)*sin(q2)) + 0.25024*cos(q2)*cos(q3)*sin(q1);
 
J2_3 = 0.14615*sin(q4)*(cos(q2)*sin(q1)*sin(q3) - 1.0*cos(q3)*sin(q1)*sin(q2)) - 0.12486*cos(q5)*(sin(q1)*sin(q2)*sin(q3) + cos(q2)*cos(q3)*sin(q1)) - 0.25024*sin(q1)*sin(q2)*sin(q3) - 0.14418*cos(q4)*sin(q5)*(cos(q2)*sin(q1)*sin(q3) - 1.0*cos(q3)*sin(q1)*sin(q2)) - 0.072089*cos(q5)*sin(q4)*(cos(q2)*sin(q1)*sin(q3) - 1.0*cos(q3)*sin(q1)*sin(q2)) - 0.25024*cos(q2)*cos(q3)*sin(q1);
 
J2_4 = 0.072089*cos(q5)*(cos(q1)*sin(q4) + cos(q4)*(sin(q1)*sin(q2)*sin(q3) + cos(q2)*cos(q3)*sin(q1))) - 0.14615*cos(q1)*sin(q4) + 0.14418*sin(q5)*(cos(q1)*cos(q4) - 1.0*sin(q4)*(sin(q1)*sin(q2)*sin(q3) + cos(q2)*cos(q3)*sin(q1))) - 0.14615*cos(q4)*(sin(q1)*sin(q2)*sin(q3) + cos(q2)*cos(q3)*sin(q1));
 
J2_5 = 0.14418*cos(q5)*(cos(q1)*sin(q4) + cos(q4)*(sin(q1)*sin(q2)*sin(q3) + cos(q2)*cos(q3)*sin(q1))) + 0.072089*sin(q5)*(cos(q1)*cos(q4) - 1.0*sin(q4)*(sin(q1)*sin(q2)*sin(q3) + cos(q2)*cos(q3)*sin(q1))) + 0.12486*sin(q5)*(cos(q2)*sin(q1)*sin(q3) - 1.0*cos(q3)*sin(q1)*sin(q2));
 
J2_6 = 0.0;
 
J3_1 = 0.0;
 
J3_2 = 0.29*sin(q2) + 0.12486*cos(q5)*(cos(q2)*sin(q3) - 1.0*cos(q3)*sin(q2)) + 0.25024*cos(q2)*sin(q3) - 0.25024*cos(q3)*sin(q2) + 0.14615*sin(q4)*(cos(q2)*cos(q3) + sin(q2)*sin(q3)) - 0.14418*cos(q4)*sin(q5)*(cos(q2)*cos(q3) + sin(q2)*sin(q3)) - 0.072089*cos(q5)*sin(q4)*(cos(q2)*cos(q3) + sin(q2)*sin(q3));
 
J3_3 = 0.25024*cos(q3)*sin(q2) - 0.25024*cos(q2)*sin(q3) - 0.12486*cos(q5)*(cos(q2)*sin(q3) - 1.0*cos(q3)*sin(q2)) - 0.14615*sin(q4)*(cos(q2)*cos(q3) + sin(q2)*sin(q3)) + 0.14418*cos(q4)*sin(q5)*(cos(q2)*cos(q3) + sin(q2)*sin(q3)) + 0.072089*cos(q5)*sin(q4)*(cos(q2)*cos(q3) + sin(q2)*sin(q3));
 
J3_4 = 0.072089*cos(q4)*cos(q5)*(cos(q2)*sin(q3) - 1.0*cos(q3)*sin(q2)) - 0.14615*cos(q4)*(cos(q2)*sin(q3) - 1.0*cos(q3)*sin(q2)) - 0.14418*sin(q4)*sin(q5)*(cos(q2)*sin(q3) - 1.0*cos(q3)*sin(q2));
 
J3_5 = 0.14418*cos(q4)*cos(q5)*(cos(q2)*sin(q3) - 1.0*cos(q3)*sin(q2)) - 0.12486*sin(q5)*(cos(q2)*cos(q3) + sin(q2)*sin(q3)) - 0.072089*sin(q4)*sin(q5)*(cos(q2)*sin(q3) - 1.0*cos(q3)*sin(q2));
 
J3_6 = 0.0;
 
J4_1 = 0.0;
 
J4_2 = -1.0*sin(q1);
 
J4_3 = sin(q1);
 
J4_4 = cos(q1)*cos(q3)*sin(q2) - 1.0*cos(q1)*cos(q2)*sin(q3);
 
J4_5 = 0.5*cos(q1)*cos(q3)*sin(q2) - 0.86603*sin(q4)*(cos(q1)*cos(q2)*cos(q3) + cos(q1)*sin(q2)*sin(q3)) - 0.5*cos(q1)*cos(q2)*sin(q3) - 0.86603*cos(q4)*sin(q1);
 
J4_6 = 0.43301*cos(q5)*(cos(q4)*sin(q1) + sin(q4)*(cos(q1)*cos(q2)*cos(q3) + cos(q1)*sin(q2)*sin(q3))) - 0.43301*cos(q4)*sin(q1) - 0.86603*sin(q5)*(sin(q1)*sin(q4) - 1.0*cos(q4)*(cos(q1)*cos(q2)*cos(q3) + cos(q1)*sin(q2)*sin(q3))) - 0.43301*sin(q4)*(cos(q1)*cos(q2)*cos(q3) + cos(q1)*sin(q2)*sin(q3)) - 0.75*cos(q5)*(cos(q1)*cos(q2)*sin(q3) - 1.0*cos(q1)*cos(q3)*sin(q2)) - 0.25*cos(q1)*cos(q2)*sin(q3) + 0.25*cos(q1)*cos(q3)*sin(q2);
 
J5_1 = 0.0;
 
J5_2 = -1.0*cos(q1);
 
J5_3 = cos(q1);
 
J5_4 = cos(q2)*sin(q1)*sin(q3) - 1.0*cos(q3)*sin(q1)*sin(q2);
 
J5_5 = 0.86603*sin(q4)*(sin(q1)*sin(q2)*sin(q3) + cos(q2)*cos(q3)*sin(q1)) - 0.86603*cos(q1)*cos(q4) + 0.5*cos(q2)*sin(q1)*sin(q3) - 0.5*cos(q3)*sin(q1)*sin(q2);
 
J5_6 = 0.43301*cos(q5)*(cos(q1)*cos(q4) - 1.0*sin(q4)*(sin(q1)*sin(q2)*sin(q3) + cos(q2)*cos(q3)*sin(q1))) - 0.86603*sin(q5)*(cos(q1)*sin(q4) + cos(q4)*(sin(q1)*sin(q2)*sin(q3) + cos(q2)*cos(q3)*sin(q1))) - 0.43301*cos(q1)*cos(q4) + 0.43301*sin(q4)*(sin(q1)*sin(q2)*sin(q3) + cos(q2)*cos(q3)*sin(q1)) + 0.75*cos(q5)*(cos(q2)*sin(q1)*sin(q3) - 1.0*cos(q3)*sin(q1)*sin(q2)) + 0.25*cos(q2)*sin(q1)*sin(q3) - 0.25*cos(q3)*sin(q1)*sin(q2);
 
J6_1 = -1.0;
 
J6_2 = 0.0;
 
J6_3 = 0.0;
 
J6_4 = - 1.0*cos(q2)*cos(q3) - 1.0*sin(q2)*sin(q3);
 
J6_5 = 0.86603*sin(q4)*(cos(q2)*sin(q3) - 1.0*cos(q3)*sin(q2)) - 0.5*cos(q2)*cos(q3) - 0.5*sin(q2)*sin(q3);
 
J6_6 = 0.43301*sin(q4)*(cos(q2)*sin(q3) - 1.0*cos(q3)*sin(q2)) - 0.25*cos(q2)*cos(q3) - 0.25*sin(q2)*sin(q3) - 0.75*cos(q5)*(cos(q2)*cos(q3) + sin(q2)*sin(q3)) - 0.86603*cos(q4)*sin(q5)*(cos(q2)*sin(q3) - 1.0*cos(q3)*sin(q2)) - 0.43301*cos(q5)*sin(q4)*(cos(q2)*sin(q3) - 1.0*cos(q3)*sin(q2));
 
 
Jac =[  J1_1, J1_2, J1_3, J1_4, J1_5, J1_6;
        J2_1, J2_2, J2_3, J2_4, J2_5, J2_6;
        J3_1, J3_2, J3_3, J3_4, J3_5, J3_6;
        J4_1, J4_2, J4_3, J4_4, J4_5, J4_6;
        J5_1, J5_2, J5_3, J5_4, J5_5, J5_6;
        J6_1, J6_2, J6_3, J6_4, J6_5, J6_6];
